simulink model "SVPWM_Close_Loop_Speed"  (R2018a)
settings: Solver=ode3  StartTime=0.0  StopTime=2  FixedStep=0.000001  RelTol=1e-3
libraries: powerlib x4, simulink x1
settings Model: Creator=Stephen  LastModifiedBy=Stephen

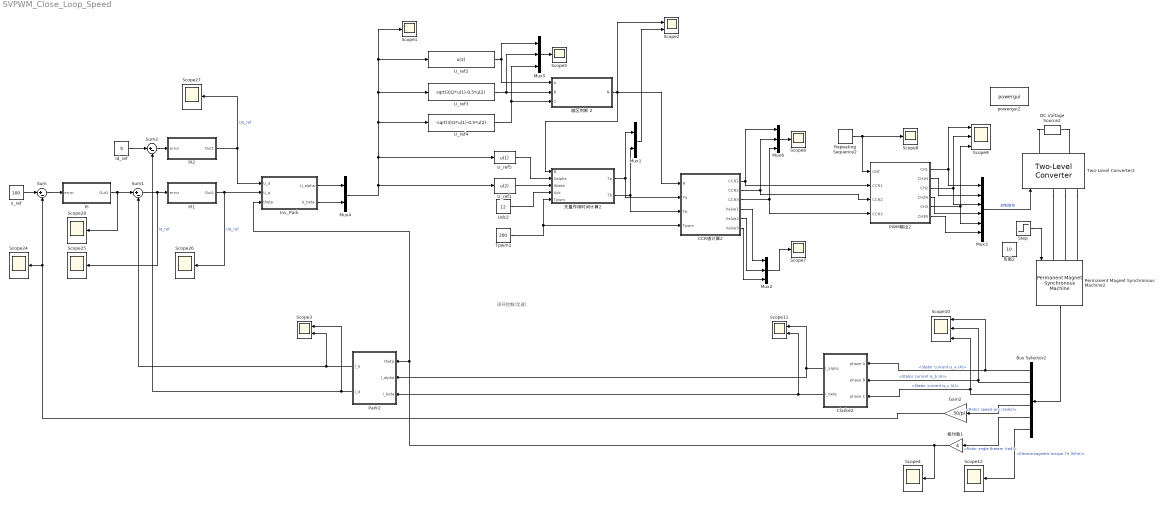
== system SVPWM_Close_Loop_Speed ==
  note: 闭环控制(定速)
  Bus Selector2 : BusSelector  OutputSignals=Stator current is_a (A),Stator current is_b (A),Stator current is_c (A),Rotor speed wm (rad/s),Rotor angle thetam (rad),Electromagnetic torque Te (N*m)
  CCR值计算2 : MATLAB Function  TreatAsAtomicUnit=on
  Clarke2 : Subsystem
  DC Voltage Source2 : powerlib/Electrical Sources/DC Voltage Source  Amplitude=12  Measurements=None
  Gain2 : Gain  Gain=30/pi
  Id_ref : Constant  Value=0
  Inv_Park : Subsystem
  Mux1 : Mux  Inputs=2
  Mux2 : Mux  Inputs=3
  Mux3 : Mux  Inputs=6
  Mux4 : Mux  Inputs=2
  Mux5 : Mux  Inputs=3
  Mux6 : Mux  Inputs=3
  PI : Subsystem
  PI1 : Subsystem
  PI2 : Subsystem
  PWM输出2 : MATLAB Function  TreatAsAtomicUnit=on
  Park2 : Subsystem
  Permanent Magnet Synchronous Machine2 : powerlib/Machines/Permanent Magnet Synchronous Machine  NbPhases=3  FluxDistribution=Sinusoidal  RotorType=Round  MechanicalLoad=Torque Tm  PresetModel=No  ShowDetailedParameters=on  MeasurementBus=off  Resistance=0.0485  Inductance=8.5e-3  dqInductances=[8.5e-3,8.5e-3]  La=0.000395  MachineConstant=Flux linkage established by magnets (V.s)  Flux=0.1194  VoltageCst=86.6271  TorqueCst=0.7164  Flat=120  Mechanical=[0.0027 0.0004924 4 0]  PolePairs=4  InitialConditions=[0,0, 0,0]  InitialConditions5ph=[0 0 0 0 0 0]  TsPowergui=0  TsBlock=-1  RefAngle=Aligned with phase A axis (original Park)
      settings: SourceProductName=Simscape Power Systems
  Repeating Sequence2 : simulink/Sources/Repeating Sequence  rep_seq_t=[0 0.00005 0.0001]  rep_seq_y=[0 100 0]
  Scope{1,4..8,12,24..28} (12 alike) : Scope
  Scope10 : Scope  NumInputPorts=3
  Scope11 : Scope  NumInputPorts=2
  Scope2 : Scope  NumInputPorts=2
  Scope3 : Scope  NumInputPorts=2
  Scope9 : Scope  NumInputPorts=3
  Step : Step  After=10  SampleTime=0
  Sum : Sum  Inputs=|+-
  Sum1 : Sum  Inputs=|+-
  Sum2 : Sum  Inputs=|+-
  Tpwm2 : Constant  Value=200
  Two-Level Converter2 : powerlib/Power Electronics/Two-Level Converter  ModelType=Switching devices  Ron=1e-3  Rs=1e6  Cs=inf  Vforward=[0,0]  Ron_Diode=1e-3  Rs_Diode=1e6  Cs_Diode=inf  Vf_Diode=1e-3  Rs_CurrentSource=inf
      settings: SourceProductName=Simscape Power Systems  SourceProductBaseCode=PS
  U_ref1 : Fcn  Expr=u(2)
  U_ref2 : Fcn  Expr=u(2)
  U_ref3 : Fcn  Expr=sqrt(3)/2*u(1)-0.5*u(2)
  U_ref4 : Fcn  Expr=-sqrt(3)/2*u(1)-0.5*u(2)
  U_ref5 : Fcn  Expr=u(1)
  Udc2 : Constant  Value=12
  n_ref : Constant  Value=100
  powergui2 : powerlib/powergui  Priority=1  SimulationMode=Discrete  SampleTime=0.000001  frequency=60  Iterations=50  frequencyindice=0  Pbase=100e6  ErrMax=1e-4  UnitsV=kV  UnitsW=MW  buscounter=0  FunctionMessages=off  echomessages=off  EnableUseOfTLC=off  CurrentSourceSwitches=off  DisableSnubberDevices=off  DisableRonSwitches=off  DisableVfSwitches=off  DisplayEquations=off  SolverType=Tustin/Backward Euler (TBE)  Interpol=off  ExternalGateDelay=off  methode=off  Ts=100  x0status=blocks  SPID=on  SwTol=0  HookPort=off  RestoreLinks=warning  ResistiveCurrentMeasurement=off  Frange=[0:2:500]  Ylog=off  Xlog=on  ShowGrid=off  save=off  variable=ZData  structure=0  ZoomFFT=off  StartTime=0.0  cycles=1  DisplayStyle=1  fundamental=60  FreqAxis=off  MaxFrequency=1000  frequencyindicesteady=1  RmsSteady=1  display=off
  扇区判断 2 : MATLAB Function  TreatAsAtomicUnit=on
  极对数1 : Gain  Gain=4
  矢量作用时间计算2 : MATLAB Function  TreatAsAtomicUnit=on
  负载2 : Constant  Value=10
  wires:
  Sum2/1 -> PI2/1("error ")
  Park2/2(I_d) -> Scope3/1, Sum2/2
  PI2/1(Out1) -> Scope27/1, Inv_Park/1(U_d)  "Ud_ref"
  Permanent Magnet Synchronous Machine2/1 -> Bus Selector2/1
  PI1/1(Out1) -> Scope26/1, Inv_Park/2(U_q)  "Uq_ref"
  Sum1/1 -> Scope25/1, PI1/1("error ")  "Iq_ref"
  PWM输出2/2(CH1N) -> Mux3/2
  CCR值计算2/4(Value1) -> Mux2/1
  PI/1(Out1) -> Scope28/1, Sum1/1
  Gain2/1 -> Sum/2, Scope24/1
  Id_ref/1 -> Sum2/1
  Tpwm2/1 -> CCR值计算2/4(Tpwm), 矢量作用时间计算2/5(Tpwm)
  U_ref5/1 -> 矢量作用时间计算2/2(Ualpha)
  n_ref/1 -> Sum/1
  CCR值计算2/6(Value3) -> Mux2/3
  矢量作用时间计算2/1(Ta) -> CCR值计算2/2(Ta), Mux1/1
  PWM输出2/4(CH2N) -> Mux3/4
  U_ref3/1 -> Mux5/2, 扇区判断 2/2(B)
  U_ref2/1 -> 扇区判断 2/1(A), Mux5/1
  Sum/1 -> PI/1("error ")
  Mux6/1 -> Scope6/1
  Inv_Park/2(U_beta) -> Mux4/2
  PWM输出2/6(CH3N) -> Mux3/6
  Repeating Sequence2/1 -> PWM输出2/1(CNT), Scope8/1
  Bus Selector2/1 -> Scope10/1, Clarke2/1(phase A)  "<Stator current is_a (A)>"
  Mux5/1 -> Scope5/1
  Mux1/1 -> Scope2/2
  极对数1/1 -> Park2/1(theta), Inv_Park/3(theta), Scope4/1
  PWM输出2/5(CH3) -> Mux3/5, Scope9/3
  Park2/1(I_q) -> Sum1/2, Scope3/2
  PWM输出2/3(CH2) -> Mux3/3, Scope9/2
  扇区判断 2/1(N) -> CCR值计算2/1(N), Scope2/1, 矢量作用时间计算2/1(N)
  Bus Selector2/3 -> Clarke2/3(phase C), Scope10/3  "<Stator current is_c (A)>"
  U_ref1/1 -> 矢量作用时间计算2/3(Ubeta)
  Bus Selector2/4 -> Gain2/1  "<Rotor speed wm (rad/s)>"
  PWM输出2/1(CH1) -> Mux3/1, Scope9/1
  CCR值计算2/5(Value2) -> Mux2/2
  CCR值计算2/1(CCR1) -> PWM输出2/2(CCR1), Mux6/1
  矢量作用时间计算2/2(Tb) -> CCR值计算2/3(Tb), Mux1/2
  Mux3/1 -> Two-Level Converter2/1  "控制信号"
  Mux2/1 -> Scope7/1
  U_ref4/1 -> Mux5/3, 扇区判断 2/3(C)
  CCR值计算2/3(CCR3) -> Mux6/3, PWM输出2/4(CCR3)
  Bus Selector2/2 -> Clarke2/2(phase B), Scope10/2  "<Stator current is_b (A)>"
  Udc2/1 -> 矢量作用时间计算2/4(Udc)
  Clarke2/1(I_alpha) -> Scope11/1, Park2/2(I_alpha)
  Bus Selector2/5 -> 极对数1/1  "<Rotor angle thetam (rad)>"
  Inv_Park/1(U_alpha) -> Mux4/1
  CCR值计算2/2(CCR2) -> PWM输出2/3(CCR2), Mux6/2
  Mux4/1 -> U_ref1/1, U_ref5/1, U_ref3/1, Scope1/1, U_ref2/1, U_ref4/1
  Clarke2/2(I_beta) -> Scope11/2, Park2/3(I_beta)
  Bus Selector2/6 -> Scope12/1  "<Electromagnetic torque Te (N*m)>"
  Step/1 -> Permanent Magnet Synchronous Machine2/1
  connections:
  DC Voltage Source2/LConn1 -- Two-Level Converter2/RConn2
  Two-Level Converter2/LConn2 -- Permanent Magnet Synchronous Machine2/LConn2
  Two-Level Converter2/LConn3 -- Permanent Magnet Synchronous Machine2/LConn3
  DC Voltage Source2/RConn1 -- Two-Level Converter2/RConn1
  Two-Level Converter2/LConn1 -- Permanent Magnet Synchronous Machine2/LConn1

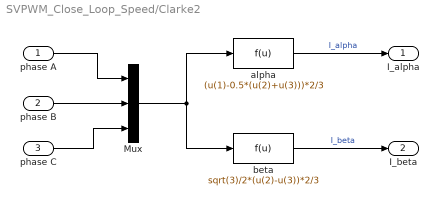
== system SVPWM_Close_Loop_Speed/Clarke2 ==
  phase A : Inport
  phase B : Inport  Port=2
  phase C : Inport  Port=3
  Mux : Mux  Inputs=3
  alpha : Fcn  Expr=(u(1)-0.5*(u(2)+u(3)))*2/3
  beta : Fcn  Expr=sqrt(3)/2*(u(2)-u(3))*2/3
  I_alpha : Outport
  I_beta : Outport  Port=2
  wires:
  Mux/1 -> alpha/1, beta/1
  alpha/1 -> I_alpha/1  "I_alpha"
  beta/1 -> I_beta/1  "I_beta"
  phase A/1 -> Mux/1
  phase B/1 -> Mux/2
  phase C/1 -> Mux/3

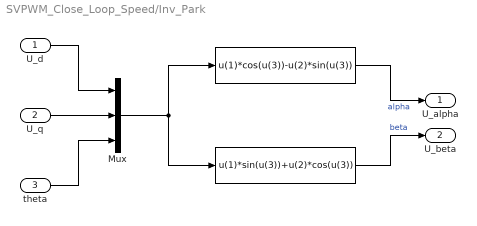
== system SVPWM_Close_Loop_Speed/Inv_Park ==
  U_d : Inport
  U_q : Inport  Port=2
  theta : Inport  Port=3
  " " : Fcn  Expr=u(1)*cos(u(3))-u(2)*sin(u(3))
  "  " : Fcn  Expr=u(1)*sin(u(3))+u(2)*cos(u(3))
  Mux : Mux  Inputs=3
  U_alpha : Outport
  U_beta : Outport  Port=2
  wires:
  "  "/1 -> U_beta/1  "beta"
  Mux/1 -> "  "/1, " "/1
  U_d/1 -> Mux/1
  theta/1 -> Mux/3
  " "/1 -> U_alpha/1  "alpha"
  U_q/1 -> Mux/2

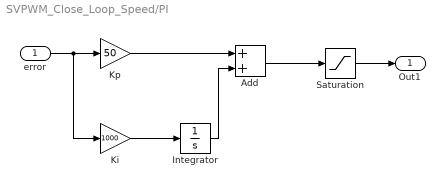
== system SVPWM_Close_Loop_Speed/PI ==
  "error " : Inport
  Add : Sum
  Integrator : Integrator
  Ki : Gain  Gain=1000
  Kp : Gain  Gain=50
  Saturation : Saturate  UpperLimit=5000  LowerLimit=-5000
  Out1 : Outport
  wires:
  "error "/1 -> Ki/1, Kp/1
  Saturation/1 -> Out1/1
  Add/1 -> Saturation/1
  Kp/1 -> Add/1
  Integrator/1 -> Add/2
  Ki/1 -> Integrator/1

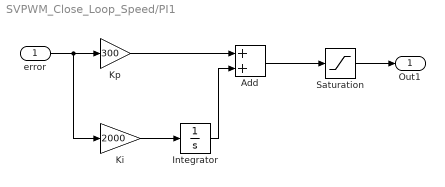
== system SVPWM_Close_Loop_Speed/PI1 ==
  "error " : Inport
  Add : Sum
  Integrator : Integrator
  Ki : Gain  Gain=2000
  Kp : Gain  Gain=300
  Saturation : Saturate  UpperLimit=7000  LowerLimit=-7000
  Out1 : Outport
  wires:
  Ki/1 -> Integrator/1
  Integrator/1 -> Add/2
  Kp/1 -> Add/1
  Add/1 -> Saturation/1
  Saturation/1 -> Out1/1
  "error "/1 -> Kp/1, Ki/1

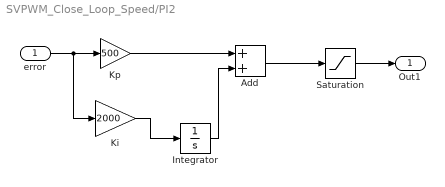
== system SVPWM_Close_Loop_Speed/PI2 ==
  "error " : Inport
  Add : Sum
  Integrator : Integrator
  Ki : Gain  Gain=2000
  Kp : Gain  Gain=500
  Saturation : Saturate  UpperLimit=10000  LowerLimit=-10000
  Out1 : Outport
  wires:
  "error "/1 -> Ki/1, Kp/1
  Saturation/1 -> Out1/1
  Add/1 -> Saturation/1
  Kp/1 -> Add/1
  Integrator/1 -> Add/2
  Ki/1 -> Integrator/1

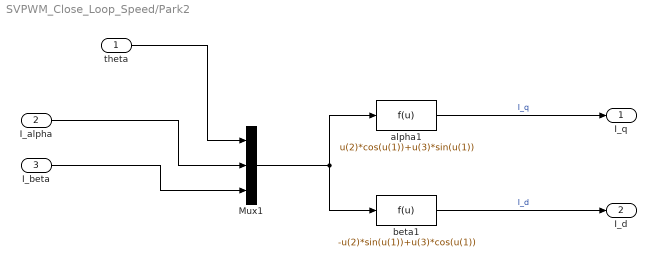
== system SVPWM_Close_Loop_Speed/Park2 ==
  theta : Inport
  I_alpha : Inport  Port=2
  I_beta : Inport  Port=3
  Mux1 : Mux  Inputs=3
  alpha1 : Fcn  Expr=u(2)*cos(u(1))+u(3)*sin(u(1))
  beta1 : Fcn  Expr=-u(2)*sin(u(1))+u(3)*cos(u(1))
  I_q : Outport
  I_d : Outport  Port=2
  wires:
  I_alpha/1 -> Mux1/2
  Mux1/1 -> beta1/1, alpha1/1
  I_beta/1 -> Mux1/3
  alpha1/1 -> I_q/1  "I_q"
  theta/1 -> Mux1/1
  beta1/1 -> I_d/1  "I_d"

== matlab function SVPWM_Close_Loop_Speed/CCR值计算2 ==
  data: N input; CCR1 output; Ta input; Tb input; Tpwm input; CCR2 output; CCR3 output; Value1 output; Value2 output; Value3 output
function [CCR1,CCR2,CCR3,Value1,Value2,Value3] = CCRCalculate(N,Ta,Tb,Tpwm)

CCR1=double(0);
CCR2=double(0);
CCR3=double(0);

Value1=(Tpwm-Ta-Tb)/4.0;
Value2=Value1+Ta/2.0;
Value3=Value2+Tb/2.0;

switch(N)
    case 3  %{扇区1 %}
        CCR1=Value1;
        CCR2=Value2;
        CCR3=Value3;

    case 1  %{扇区2%}
        CCR1=Value2;
        CCR2=Value1;
        CCR3=Value3;

    case 5  %{扇区3%}
        CCR1=Value3;
        CCR2=Value1;
        CCR3=Value2;

    case 4  %{扇区4%}
        CCR1=Value3;
        CCR2=Value2;
        CCR3=Value1;

    case 6  %{扇区5%}
        CCR1=Value2;
        CCR2=Value3;
        CCR3=Value1;

    case 2  %{扇区6%}
        CCR1=Value1;
        CCR2=Value3;
        CCR3=Value2;
end

== matlab function SVPWM_Close_Loop_Speed/PWM输出2 ==
  data: CNT input; CH1 output; CCR1 input; CCR2 input; CCR3 input; CH1N output; CH2 output; CH2N output; CH3 output; CH3N output
function [CH1,CH1N,CH2,CH2N,CH3,CH3N] = PWM(CNT,CCR1,CCR2,CCR3)

if(CNT <= CCR1)
    CH1=0;
    CH1N=1;
else
    CH1=1;
    CH1N=0;
end
if(CNT <= CCR2)
    CH2=0;
    CH2N=1;
else
    CH2=1;
    CH2N=0;
end
if(CNT <= CCR3)
    CH3=0;
    CH3N=1;
else
    CH3=1;
    CH3N=0;
end

== matlab function SVPWM_Close_Loop_Speed/扇区判断 2 ==
  data: A input; N output; B input; C input
function N = Sector_Judge(A,B,C)
N=0;

if(A>0)
    N=N+1;
end
if(B>0)
    N=N+2;
end
if(C>0)
    N=N+4;
end

== matlab function SVPWM_Close_Loop_Speed/矢量作用时间计算2 ==
  data: N input; Ta output; Ualpha input; Ubeta input; Udc input; Tpwm input; Tb output
function [Ta,Tb] = VectorCalculate(N,Ualpha,Ubeta,Udc,Tpwm)

Ta=double(0);
Tb=double(0);

X=(sqrt(3)*Tpwm)/Udc*Ubeta;
Y=(sqrt(3)*Tpwm)/Udc*((sqrt(3)/2)*Ualpha+0.5*Ubeta);
Z=(sqrt(3)*Tpwm)/Udc*(-(sqrt(3)/2)*Ualpha+0.5*Ubeta);

if(N==3)  %{扇区1 %}
    Ta=-Z;
    Tb=X;
end
if(N==1)  %{扇区2%}
    Ta=Z;
    Tb=Y;
end
if(N==5)  %{扇区3%}
    Ta=X;
    Tb=-Y;
end
if(N==4)  %{扇区4%}
    Ta=-X;
    Tb=Z;
end
if(N==6)  %{扇区5%}
    Ta=-Y;
    Tb=-Z;
end
if(N==2)  %{扇区6%}
    Ta=Y;
    Tb=-X;
end
Tsum = Ta+Tb;
if(Tsum>Tpwm)  %过调制
    Ta=Tpwm*Ta/Tsum;
    Tb=Tpwm*Tb/Tsum;
end
